simulink model "solar_wind_system_with_statcom"  (R2024a)
settings: Solver=VariableStepAuto  StartTime=0.0  StopTime=1  RelTol=1e-3
undefined symbols (not defined in the file): DiscIntNeverNeededParam, R
libraries: neural x24, spsSeriesRLCBranchLib x24, spsVoltageMeasurementLib x12, spsDiodeLib x10, powerlib_extras x9, simulink x7, spsIGBTDiodeLib x6, spsCurrentMeasurementLib x5, spsThreePhaseVIMeasurementLib x4, spsBreakerLib x3, spsPower3phInstantaneousLib x3, spsControlledCurrentSourceLib x3
(part 1 of 3)
settings Model: Creator=prabh  LastModifiedBy=HP

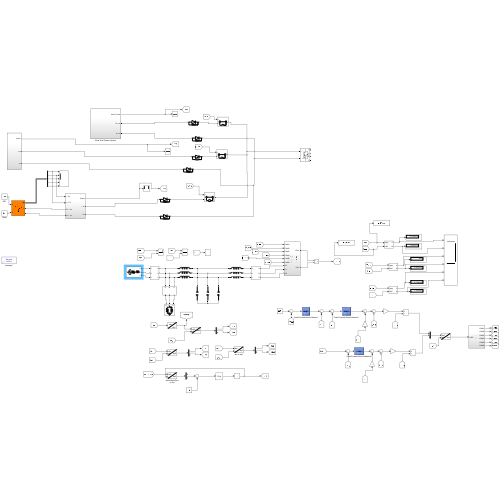
[thumbnail: Simulink's stored preview of the top-level diagram]
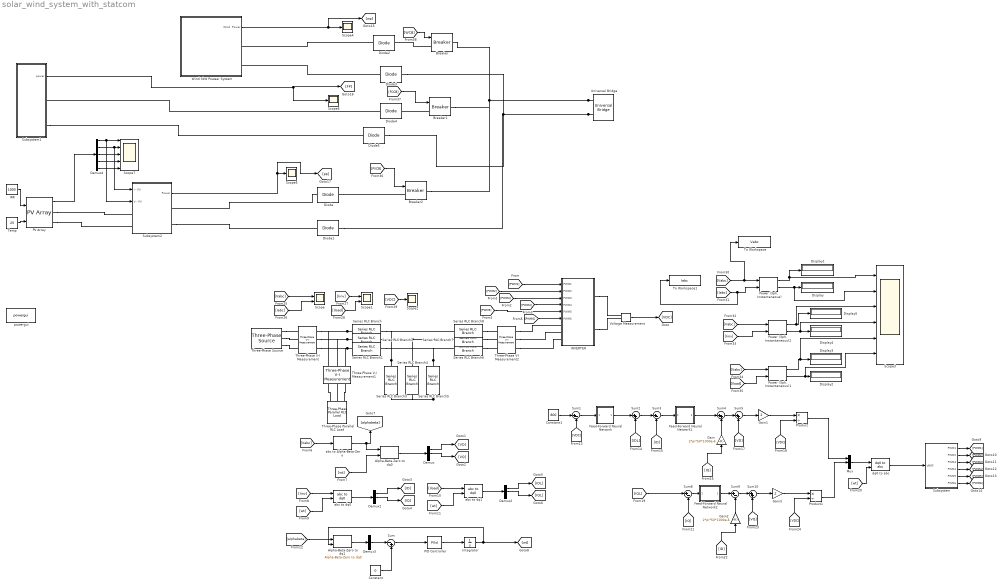
== system solar_wind_system_with_statcom ==
  Alpha-Beta-Zero to dq0 : spsAlphaBetaZerotodq0Lib/Alpha-Beta-Zero to dq0  Alignment=90 degrees behind phase A axis
  Alpha-Beta-Zero to dq1 : spsAlphaBetaZerotodq0Lib/Alpha-Beta-Zero to dq0  Alignment=90 degrees behind phase A axis
  Breaker : spsBreakerLib/Breaker  InitialState=1  SwitchingTimes="[1/60  5/60]"  External=on  BreakerResistance=0.01  SnubberResistance=1e6  SnubberCapacitance=inf  Measurements=None  MoreParameters=on  NoBreakLoop=off
  Breaker1 : spsBreakerLib/Breaker  InitialState=1  SwitchingTimes="[1/60  5/60]"  External=on  BreakerResistance=0.01  SnubberResistance=1e6  SnubberCapacitance=inf  Measurements=None  MoreParameters=on  NoBreakLoop=off
  Breaker2 : spsBreakerLib/Breaker  InitialState=1  SwitchingTimes="[1/60  5/60]"  External=on  BreakerResistance=0.01  SnubberResistance=1e6  SnubberCapacitance=inf  Measurements=None  MoreParameters=on  NoBreakLoop=off
  Constant : Constant  Value=0
  Constant1 : Constant  Value=800
  Demux{,1..3} (4 alike) : Demux  Outputs=3
  Demux4 : Demux  Outputs=5
  Diode{,1..5} (6 alike) : spsDiodeLib/Diode  Ron=0.001  Lon=0  Vf=0.8  IC=0  UseSnubber=off  Rs=500  Cs=250e-9  Measurements=off
  Display{,1..5} (6 alike) : Display
  Feed-Forward Neural Network : Subsystem
      mask help: Feed-Forward Neural Network
      mask Display: e = 0.06;c1 = [120 150 230]/255;c2 = ([120 150 230]+0)/383;c3 = ([120 150 230]+128)/383;patch([0 1 1 0],[0 0 1 1],c1);patch([0 1 1 1-e 1-e 0+e],[0 0 1 1-e 0+e 0+e],c2);patch([0 0 1 1-e 0+e 0+e],[0 1 1 1-e 1-e 0+e],c3);plot([0 1 1 0 0],[0 0 1 1 0]);fprintf('NNET');port_label('input',1,' Input');port_label('output',1,'Output ');
  Feed-Forward Neural Network1 : Subsystem
      mask help: Feed-Forward Neural Network
      mask Display: e = 0.06;c1 = [120 150 230]/255;c2 = ([120 150 230]+0)/383;c3 = ([120 150 230]+128)/383;patch([0 1 1 0],[0 0 1 1],c1);patch([0 1 1 1-e 1-e 0+e],[0 0 1 1-e 0+e 0+e],c2);patch([0 0 1 1-e 0+e 0+e],[0 1 1 1-e 1-e 0+e],c3);plot([0 1 1 0 0],[0 0 1 1 0]);fprintf('NNET');port_label('input',1,' Input');port_label('output',1,'Output ');
  Feed-Forward Neural Network2 : Subsystem
      mask help: Feed-Forward Neural Network
      mask Display: e = 0.06;c1 = [120 150 230]/255;c2 = ([120 150 230]+0)/383;c3 = ([120 150 230]+128)/383;patch([0 1 1 0],[0 0 1 1],c1);patch([0 1 1 1-e 1-e 0+e],[0 0 1 1-e 0+e 0+e],c2);patch([0 0 1 1-e 0+e 0+e],[0 1 1 1-e 1-e 0+e],c3);plot([0 1 1 0 0],[0 0 1 1 0]);fprintf('NNET');port_label('input',1,' Input');port_label('output',1,'Output ');
  Gain : Gain  Gain=2*pi*50*1000e-6
  Gain1 : Gain  Gain=2
  Gain2 : Gain  Gain=2*pi*50*1000e-6
  Gain3 : Gain  Gain=2
  INVERTER : Subsystem
  IRR : Constant  Value=1000
  Integrator : Integrator
  Mux : Mux  Inputs=3
  PID Controller : slpidlib/PID Controller  Controller=PI  Form=Parallel  TimeDomain=Continuous-time  UseExternalTs=off  SampleTime=-1  IntegratorMethod=Forward Euler  FilterMethod=Forward Euler  ControllerParametersSource=internal  P=10  I=50000  UseKiTs=off  D=0  UseExternalDerivativeSource=off  N=100  UseFilter=on  TunerSelectOption=Transfer Function Based (PID Tuner App)  InitialConditionSource=internal  InitialConditionForIntegrator=0  InitialConditionForFilter=0  DifferentiatorICPrevScaledInput=0  ExternalReset=none  TrackingMode=off  Kt=1  LimitOutput=off  SatLimitsSource=internal  UpperSaturationLimit=inf  LowerSaturationLimit=-inf  LinearizeAsGain=on  AntiWindupMode=none  Kb=1  LimitIntegrator=off  UpperIntegratorSaturationLimit=inf  LowerIntegratorSaturationLimit=-inf  POutMin=[]  POutMax=[]  IOutMin=[]  IOutMax=[]  DOutMin=[]  DOutMax=[]  NOutMin=[]  NOutMax=[]  SumOutMin=[]  SumOutMax=[]  SaturationOutMin=[]  SaturationOutMax=[]  PParamMin=[]  PParamMax=[]  IParamMin=[]  IParamMax=[]  DParamMin=[]  DParamMax=[]  NParamMin=[]  NParamMax=[]  KbParamMin=[]  KbParamMax=[]  KtParamMin=[]  KtParamMax=[]  KbOutMin=[]  KbOutMax=[]  KtOutMin=[]  KtOutMax=[]  IntegratorOutMin=[]  IntegratorOutMax=[]  FilterOutMin=[]  FilterOutMax=[]  SumI1OutMin=[]  SumI1OutMax=[]  SumI2OutMin=[]  SumI2OutMax=[]  SumI3OutMin=[]  SumI3OutMax=[]  SumI4OutMin=[]  SumI4OutMax=[]  SumDOutMin=[]  SumDOutMax=[]  DifferentiatorOutMin=[]  DifferentiatorOutMax=[]  FilterDiffOutCoefMin=[]  FilterDiffOutCoefMax=[]  ReciprocalOutMin=[]  ReciprocalOutMax=[]  SumDenOutMin=[]  SumDenOutMax=[]  SumNumOutMin=[]  SumNumOutMax=[]  DivideOutMin=[]  DivideOutMax=[]  UdiffTsProdOutMin=[]  UdiffTsProdOutMax=[]  NTsProdOutMin=[]  NTsProdOutMax=[]  UintegralTsProdOutMin=[]  UintegralTsProdOutMax=[]  UngainTsProdOutMin=[]  UngainTsProdOutMax=[]  ClampingZeroOutDataTypeStr=Inherit: Inherit via back propagation  ClampingZeroOutMin=[]  ClampingZeroOutMax=[]  FilterDenConstantOutDataTypeStr=Inherit: Inherit via back propagation  FilterDenConstantOutMin=[]  FilterDenConstantOutMax=[]  PCopyOutDataTypeStr=Inherit: Inherit via back propagation  PCopyOutMin=[]  PCopyOutMax=[]  NCopyOutDataTypeStr=Inherit: Inherit via back propagation  NCopyOutMin=[]  NCopyOutMax=[]  IntegratorContinuousStateAttributes=''  IntegratorStateMustResolveToSignalObject=off  IntegratorRTWStateStorageClass=Auto  FilterContinuousStateAttributes=''  FilterStateMustResolveToSignalObject=off  FilterRTWStateStorageClass=Auto  ParallelPVariant=InternalParameters  IdealPVariant=Disabled  IVariant=InternalParameters  DVariant=Disabled  IntegratorVariant=Continuous  SatVariant=Disabled  AWVariant=Passthrough  PCopyVariant=Disabled  TRVariant=Disabled  FdbkBlocksVariant=Forward  IdealPFdbkVariant=Disabled  SatFdbkVariant=Disabled  DerivativeFilterVariant=Disabled  NVariant=Disabled  NCopyVariant=Disabled_SignalSpec  FilterICVariant=Disabled  IntegratorICVariant=InternalICs  ExternalResetVariant=Disabled  TRSumVariant=Passthrough  SumFdbkVariant=Disabled  SumVariant=Sum_PI  TsampFilterVariant=InternalTs  TsampNgainVariant=Passthrough  TsampIntegralVariant=Disabled_SignalSpec  ExternalSaturationOutDataTypeStr=Inherit: Same as second input  DerivativeSourceVariant=Disabled
  PV Array : spsPVArrayLib/PV Array  Npar=10  Nser=5  PlotType=array @ 25 deg.C & specified irradiances  S_vec="[ 1000  500  100 ]"  Temp_C_vec="[ 45 25  ]"  ModuleName=User-defined  PlotWhenSelected=off  Pm=334.905  Ncell=80  Voc=49.9  Isc=9  Vm=41.5  Im=8.07  beta_Voc_pc=-0.36  alpha_Isc_pc=0.09  beta_Voc=-0.17964  alpha_Isc=0.0081  IL=9.0297  I0=3.1312e-10  nI=1.0111  Rsh=77.6407  Rs=0.25633  RobustModel=off  RobustCellTemperature=313.3991  BAL=off  Tc=1e-6  Tfilter=5e-5
  "Power (3ph, Instantaneous)" : spsPower3phInstantaneousLib/Power (3ph, Instantaneous)
  "Power (3ph, Instantaneous)1" : spsPower3phInstantaneousLib/Power (3ph, Instantaneous)
  "Power (3ph, Instantaneous)2" : spsPower3phInstantaneousLib/Power (3ph, Instantaneous)
  Product : Product  Inputs=*/
  Product1 : Product  Inputs=*/
  Scope : Scope  NumInputPorts=2
  Scope1 : Scope  NumInputPorts=2
  Scope{2,4..6} (4 alike) : Scope
  Scope3 : Scope  NumInputPorts=6
  Scope7 : Scope  NumInputPorts=5
  Series RLC Branch{,1..2,6..8} (6 alike) : spsSeriesRLCBranchLib/Series RLC Branch  LConnTagsString=__new0  RConnTagsString=__new0  BranchType=L  Resistance=1  Inductance=500e-6  SetiL0=off  InitialCurrent=0  Capacitance=1e-6  Setx0=off  InitialVoltage=0  Measurements=None
  Series RLC Branch3 : spsSeriesRLCBranchLib/Series RLC Branch  LConnTagsString=__new0  RConnTagsString=__new0  BranchType=C  Resistance=1  Inductance=500e-6  SetiL0=off  InitialCurrent=0  Capacitance=100e-6  Setx0=off  InitialVoltage=0  Measurements=None
  Series RLC Branch4 : spsSeriesRLCBranchLib/Series RLC Branch  LConnTagsString=__new0  RConnTagsString=__new0  BranchType=C  Resistance=1  Inductance=500e-6  SetiL0=off  InitialCurrent=0  Capacitance=100e-6  Setx0=off  InitialVoltage=0  Measurements=None
  Series RLC Branch5 : spsSeriesRLCBranchLib/Series RLC Branch  LConnTagsString=__new0  RConnTagsString=__new0  BranchType=C  Resistance=1  Inductance=500e-6  SetiL0=off  InitialCurrent=0  Capacitance=100e-6  Setx0=off  InitialVoltage=0  Measurements=None
  Subsystem : Subsystem
  Subsystem1 : Subsystem
  Subsystem2 : Subsystem
  Sum : Sum  Inputs=|-+
  Sum{1,3,8..9} (4 alike) : Sum  Inputs=|+-
  Sum{2,4..5,10} (4 alike) : Sum  Inputs=|++
  "Temp " : Constant  Value=25
  Three-Phase Parallel RLC Load : spsThreePhaseParallelRLCLoadLib/Three-Phase Parallel RLC Load  LConnTagsString=A|B|C  Configuration=Y (grounded)  NominalVoltage=415  Vabc=[1e3 1e3 1e3]  Vabcp=[1e3 1e3 1e3]  NominalFrequency=50  UnbalancedPower=off  ActivePower=150000  InductivePower=75000  CapacitivePower=0  Pabc=[10e3 9e3 11e3]  QLabc=[100 90 110]  QCabc=[100 90 110]  Pabcp=[10e3 9e3 11e3]  QLabcp=[100 90 110]  QCabcp=[100 90 110]  Measurements=None  LoadType=constant Z
  Three-Phase V-I Measurement : spsThreePhaseVIMeasurementLib/Three-Phase V-I Measurement  VoltageMeasurement=phase-to-ground  SetLabelV=on  LabelV=Vabc  Vpu=off  VpuLL=off  CurrentMeasurement=yes  SetLabelI=on  LabelI=Iabc  Ipu=off  Pbase=100e6  Vbase=500e3  OutputType=Complex  PhasorSimulation=off  PSBequivalent=0
  Three-Phase V-I Measurement1 : spsThreePhaseVIMeasurementLib/Three-Phase V-I Measurement  VoltageMeasurement=phase-to-ground  SetLabelV=on  LabelV=Vload  Vpu=off  VpuLL=off  CurrentMeasurement=yes  SetLabelI=on  LabelI=Iload  Ipu=off  Pbase=100e6  Vbase=500e3  OutputType=Complex  PhasorSimulation=off  PSBequivalent=0
  Three-Phase V-I Measurement2 : spsThreePhaseVIMeasurementLib/Three-Phase V-I Measurement  VoltageMeasurement=phase-to-ground  SetLabelV=on  LabelV=Vinv  Vpu=off  VpuLL=off  CurrentMeasurement=yes  SetLabelI=on  LabelI=Iinv  Ipu=off  Pbase=100e6  Vbase=500e3  OutputType=Complex  PhasorSimulation=off  PSBequivalent=0
  Three-Phase Source : spsThreePhaseSourceLib/Three-Phase Source  InternalConnection=Y  VoltagePhases=off  Voltage=500  PhaseAngle=0  Voltage_phases=[25e3 25e3 25e3]/sqrt(3)  PhaseAngles_phases=[0 -120 +120]  Frequency=50  NonIdealSource=on  SpecifyImpedance=off  Resistance=1e-6  Inductance=1e-6  ShortCircuitLevel=100e6  BaseVoltage=415  XRratio=7  BusType=swing  Pref=10e3  Qref=0  Prefabc=[10e3, 10e3, 10e3]  Qrefabc=[0, 0, 0]  Qmin=-inf  Qmax=inf
  To Workspace : ToWorkspace  VariableName=Vabc  SampleTime=-1
  To Workspace1 : ToWorkspace  VariableName=Iabc  SampleTime=-1
  Universal Bridge : spsUniversalBridgeLib/Universal Bridge  Arms=3  SnubberResistance=1e5  SnubberCapacitance=inf  Device=MOSFET / Diodes  Ron=1e-3  Lon=0  ForwardVoltages="[  0  0  ]"  ForwardVoltage=0  GTOparameters=[ 10e-6 , 20e-6 ]  IGBTparameters=[ 1e-6 , 2e-6 ]  Measurements=None  Measurements_2=None  converterType=Rectifier
  Voltage Measurement : spsVoltageMeasurementLib/Voltage Measurement  PhasorSimulation=off  OutputType=Complex  PSBequivalent=0
  Wind 3kW Poweer System : Subsystem
  abc to Alpha-Beta-Zero : spsabctoAlphaBetaZeroLib/abc to Alpha-Beta-Zero
  abc to dq0 : spsabctodq0Lib/abc to dq0  Alignment=90 degrees behind phase A axis
  abc to dq1 : spsabctodq0Lib/abc to dq0  Alignment=90 degrees behind phase A axis
  dq0 to abc : spsdq0toabcLib/dq0 to abc  Alignment=90 degrees behind phase A axis
  powergui : sps_lib/powergui  Priority=1  SimulationMode=Discrete  SampleTime=1e-6  frequency=60  Iterations=50  frequencyindice=0  Pbase=100e6  ErrMax=1e-4  UnitsV=kV  UnitsW=MW  buscounter=0  FunctionMessages=off  echomessages=off  EnableUseOfTLC=off  CurrentSourceSwitches=off  DisableSnubberDevices=off  DisableRonSwitches=off  DisableVfSwitches=off  DisplayEquations=off  AutomaticDiscreteSolvers=off  SolverType=Tustin/Backward Euler (TBE)  Interpol=off  ExternalGateDelay=off  methode=off  Ts=100  x0status=blocks  SPID=on  SwTol=0  HookPort=off  NonlinearTolerance=1e-4  nMaxIteration=100  ContinueOnMaxIteration=off  RestoreLinks=warning  ResistiveCurrentMeasurement=off  Frange=[0:2:500]  Ylog=off  Xlog=on  ShowGrid=off  save=off  variable=ZData  structure=0  ZoomFFT=off  StartTime=0.0  cycles=1  DisplayStyle=1  fundamental=60  FreqAxis=off  MaxFrequency=1000  frequencyindicesteady=1  RmsSteady=1  display=off
  wires:
  [Iload] -> "Power (3ph, Instantaneous)1"/2
  [PWM3] -> INVERTER/3(PWM3)
  [Vabc] -> "Power (3ph, Instantaneous)1"/1
  [Iload] -> Scope1/2
  Sum1/1 -> Feed-Forward Neural Network/1(Input)
  [IQL] -> Sum8/1
  [Iabc] -> To Workspace1/1, "Power (3ph, Instantaneous)"/2
  Demux2/2 -> [IQL]
  "Power (3ph, Instantaneous)2"/1 -> Scope3/3, Display5/1
  "Power (3ph, Instantaneous)1"/2 -> Scope3/6, Display2/1
  Integrator/1 -> Alpha-Beta-Zero to dq1/2, [wt]
  Sum3/1 -> Feed-Forward Neural Network1/1(Input)
  [Iinv] -> "Power (3ph, Instantaneous)2"/2
  Demux3/2 -> Sum/1
  "Power (3ph, Instantaneous)2"/2 -> Scope3/4, Display4/1
  [Iinv] -> Scope1/1
  Demux/2 -> [VQ]
  abc to Alpha-Beta-Zero/1 -> [alphabeta], Alpha-Beta-Zero to dq0/1
  [Vabc] -> To Workspace/1, "Power (3ph, Instantaneous)"/1
  "Power (3ph, Instantaneous)"/1 -> Scope3/1, Display1/1
  Alpha-Beta-Zero to dq1/1 -> Demux3/1
  Subsystem/6(PWM6) -> [PWM6]
  Demux1/2 -> [IQ]
  Subsystem/3(PWM3) -> [PWM3]
  Feed-Forward Neural Network2/1(Output) -> Sum9/1
  [Iinv] -> abc to dq0/1
  Subsystem/1(PWM1) -> [PWM1]
  [IQ] -> Sum8/2
  [Iabc] -> Scope/2
  Gain/1 -> Sum4/2
  Sum/1 -> PID Controller/1
  Subsystem/4(PWM4) -> [PWM4]
  [wt] -> dq0 to abc/2
  Voltage Measurement/1 -> [VDC]
  [VDC] -> Scope2/1
  Sum8/1 -> Feed-Forward Neural Network2/1(Input)
  [Vabc] -> Scope/1
  Mux/1 -> dq0 to abc/1
  Sum4/1 -> Sum5/1
  Product1/1 -> Mux/2
  Gain2/1 -> Sum9/2
  Sum9/1 -> Sum10/1
  Product/1 -> Mux/1
  [VQ] -> Sum10/2
  [ID] -> Sum3/2
  Gain1/1 -> Product/1
  [VD] -> Sum5/2
  Sum5/1 -> Gain1/1
  [alphabeta] -> Alpha-Beta-Zero to dq1/1
  Subsystem/2(PWM2) -> [PWM2]
  Sum2/1 -> Sum3/1
  [IQ] -> Gain/1
  [IDL] -> Sum2/2
  Gain3/1 -> Product1/1
  [Iload] -> abc to dq1/1
  [VDC] -> Sum1/2
  [Vabc] -> abc to Alpha-Beta-Zero/1
  PID Controller/1 -> Integrator/1
  [PWM5] -> INVERTER/5(PWM5)
  Subsystem/5(PWM5) -> [PWM5]
  [wt] -> abc to dq1/2
  [PWM2] -> INVERTER/2(PWM2)
  Demux1/1 -> [ID]
  [wt] -> abc to dq0/2
  [ID] -> Gain2/1
  [PWM1] -> INVERTER/1(PWM1)
  [wt] -> Alpha-Beta-Zero to dq0/2
  [VDC] -> Product1/2
  Demux2/1 -> [IDL]
  abc to dq0/1 -> Demux1/1
  dq0 to abc/1 -> Subsystem/1(VREF)
  Constant1/1 -> Sum1/1
  Alpha-Beta-Zero to dq0/1 -> Demux/1
  [PWM6] -> INVERTER/6(PWM6)
  Sum10/1 -> Gain3/1
  [Vabc] -> "Power (3ph, Instantaneous)2"/1
  "Power (3ph, Instantaneous)1"/1 -> Scope3/5, Display3/1
  [VDC] -> Product/2
  Feed-Forward Neural Network/1(Output) -> Sum2/1
  abc to dq1/1 -> Demux2/1
  Feed-Forward Neural Network1/1(Output) -> Sum4/1
  "Power (3ph, Instantaneous)"/2 -> Scope3/2, Display/1
  [PWM4] -> INVERTER/4(PWM4)
  Constant/1 -> Sum/2
  Demux/1 -> [VD]
  "Temp "/1 -> PV Array/2
  [PVCB] -> Breaker2/1
  Demux4/4 -> Scope7/4
  Subsystem1/1(power) -> [FP], Scope6/1
  Wind 3kW Poweer System/1(Wind  Power) -> [wp], Scope4/1
  Demux4/2 -> Scope7/2, Subsystem2/1(I - PV)
  IRR/1 -> PV Array/1
  [WCB] -> Breaker/1
  Subsystem2/1(Power) -> [pp], Scope5/1
  Demux4/1 -> Scope7/1, Subsystem2/2(V - PV)
  Demux4/5 -> Scope7/5
  Demux4/3 -> Scope7/3
  PV Array/1 -> Demux4/1
  [FCCB] -> Breaker1/1
  connections:
  Series RLC Branch2/LConn1 -- Three-Phase V-I Measurement/RConn3 -- Three-Phase V-I Measurement1/LConn3
  Series RLC Branch5/RConn1 -- Series RLC Branch3/RConn1 -- Series RLC Branch4/RConn1
  Series RLC Branch3/LConn1 -- Series RLC Branch8/LConn1 -- Series RLC Branch/RConn1
  Series RLC Branch7/LConn1 -- Series RLC Branch1/RConn1 -- Series RLC Branch4/LConn1
  Series RLC Branch1/LConn1 -- Three-Phase V-I Measurement/RConn2 -- Three-Phase V-I Measurement1/LConn2
  Series RLC Branch/LConn1 -- Three-Phase V-I Measurement/RConn1 -- Three-Phase V-I Measurement1/LConn1
  Series RLC Branch5/LConn1 -- Series RLC Branch6/LConn1 -- Series RLC Branch2/RConn1
  Three-Phase V-I Measurement2/LConn2 -- INVERTER/LConn2
  Series RLC Branch6/RConn1 -- Three-Phase V-I Measurement2/RConn3
  Three-Phase V-I Measurement2/LConn3 -- INVERTER/LConn3
  Three-Phase Source/RConn1 -- Three-Phase V-I Measurement/LConn1
  INVERTER/RConn2 -- Voltage Measurement/LConn2
  Three-Phase Parallel RLC Load/LConn2 -- Three-Phase V-I Measurement1/RConn2
  Series RLC Branch8/RConn1 -- Three-Phase V-I Measurement2/RConn1
  Three-Phase Parallel RLC Load/LConn3 -- Three-Phase V-I Measurement1/RConn3
  Series RLC Branch7/RConn1 -- Three-Phase V-I Measurement2/RConn2
  INVERTER/RConn1 -- Voltage Measurement/LConn1
  Three-Phase Parallel RLC Load/LConn1 -- Three-Phase V-I Measurement1/RConn1
  Three-Phase Source/RConn2 -- Three-Phase V-I Measurement/LConn2
  Three-Phase Source/RConn3 -- Three-Phase V-I Measurement/LConn3
  Three-Phase V-I Measurement2/LConn1 -- INVERTER/LConn1
  Universal Bridge/RConn2 -- Diode3/RConn1 -- Diode5/RConn1 -- Diode1/RConn1
  Universal Bridge/RConn1 -- Breaker/RConn1 -- Breaker2/RConn1 -- Breaker1/RConn1
  Diode2/LConn1 -- Wind 3kW Poweer System/RConn1
  Subsystem2/RConn2 -- Diode1/LConn1
  Subsystem1/RConn2 -- Diode5/LConn1
  PV Array/RConn1 -- Subsystem2/LConn1
  Breaker2/LConn1 -- Diode/RConn1
  Diode4/LConn1 -- Subsystem1/RConn1
  Breaker/LConn1 -- Diode2/RConn1
  Breaker1/LConn1 -- Diode4/RConn1
  PV Array/RConn2 -- Subsystem2/LConn2
  Diode3/LConn1 -- Wind 3kW Poweer System/RConn2
  Diode/LConn1 -- Subsystem2/RConn1

== system solar_wind_system_with_statcom/Feed-Forward Neural Network ==
  Input : Inport  PortDimensions=1
      mask Display: e = 0.06;c1 = [120 230 180]/255;c2 = ([120 230 180]+0)/(256+128);c3 = ([120 230 180]+128)/(256+128);patch([0 1 1 0],[0 0 1 1],c1);patch([0 1 1 1-e 1-e 0+e],[0 0 1 1-e 0+e 0+e],c2);patch([0 0 1 1-e 0+e 0+e],[0 1 1 1-e 1-e 0+e],c3);plot([0 1 1 0 0],[0 0 1 1 0]);
  Layer 1 : Subsystem
      mask Display: e = 0.06;c1 = [120 150 230]/255;c2 = ([120 150 230]+0)/383;c3 = ([120 150 230]+128)/383;patch([0 1 1 0],[0 0 1 1],c1);patch([0 1 1 1-e 1-e 0+e],[0 0 1 1-e 0+e 0+e],c2);patch([0 0 1 1-e 0+e 0+e],[0 1 1 1-e 1-e 0+e],c3);plot([0 1 1 0 0],[0 0 1 1 0]);
  Layer 2 : Subsystem
      mask Display: e = 0.06;c1 = [120 150 230]/255;c2 = ([120 150 230]+0)/383;c3 = ([120 150 230]+128)/383;patch([0 1 1 0],[0 0 1 1],c1);patch([0 1 1 1-e 1-e 0+e],[0 0 1 1-e 0+e 0+e],c2);patch([0 0 1 1-e 0+e 0+e],[0 1 1 1-e 1-e 0+e],c3);plot([0 1 1 0 0],[0 0 1 1 0]);
  Process Input 1 : Subsystem
      mask Display: e = 0.06;c1 = [120 150 230]/255;c2 = ([120 150 230]+0)/383;c3 = ([120 150 230]+128)/383;patch([0 1 1 0],[0 0 1 1],c1);patch([0 1 1 1-e 1-e 0+e],[0 0 1 1-e 0+e 0+e],c2);patch([0 0 1 1-e 0+e 0+e],[0 1 1 1-e 1-e 0+e],c3);plot([0 1 1 0 0],[0 0 1 1 0]);
  Process Output 1 : Subsystem
      mask Display: e = 0.06;c1 = [120 150 230]/255;c2 = ([120 150 230]+0)/383;c3 = ([120 150 230]+128)/383;patch([0 1 1 0],[0 0 1 1],c1);patch([0 1 1 1-e 1-e 0+e],[0 0 1 1-e 0+e 0+e],c2);patch([0 0 1 1-e 0+e 0+e],[0 1 1 1-e 1-e 0+e],c3);plot([0 1 1 0 0],[0 0 1 1 0]);
  Output : Outport  InitialOutput=0
      mask Display: e = 0.06;c1 = [120 230 180]/255;c2 = ([120 230 180]+0)/(256+128);c3 = ([120 230 180]+128)/(256+128);patch([0 1 1 0],[0 0 1 1],c1);patch([0 1 1 1-e 1-e 0+e],[0 0 1 1-e 0+e 0+e],c2);patch([0 0 1 1-e 0+e 0+e],[0 1 1 1-e 1-e 0+e],c3);plot([0 1 1 0 0],[0 0 1 1 0]);
  wires:
  Input/1 -> Process Input 1/1(x)
  Process Output 1/1(y) -> Output/1
  Process Input 1/1(p) -> Layer 1/1("p{1}")
  Layer 1/1("a{1}") -> [feedback1]
  [feedback1] -> Layer 2/1("a{1} ")
  Layer 2/1("a{2}") -> Process Output 1/1(a)

== system solar_wind_system_with_statcom/Feed-Forward Neural Network1 ==
  Input : Inport  PortDimensions=1
      mask Display: e = 0.06;c1 = [120 230 180]/255;c2 = ([120 230 180]+0)/(256+128);c3 = ([120 230 180]+128)/(256+128);patch([0 1 1 0],[0 0 1 1],c1);patch([0 1 1 1-e 1-e 0+e],[0 0 1 1-e 0+e 0+e],c2);patch([0 0 1 1-e 0+e 0+e],[0 1 1 1-e 1-e 0+e],c3);plot([0 1 1 0 0],[0 0 1 1 0]);
  Layer 1 : Subsystem
      mask Display: e = 0.06;c1 = [120 150 230]/255;c2 = ([120 150 230]+0)/383;c3 = ([120 150 230]+128)/383;patch([0 1 1 0],[0 0 1 1],c1);patch([0 1 1 1-e 1-e 0+e],[0 0 1 1-e 0+e 0+e],c2);patch([0 0 1 1-e 0+e 0+e],[0 1 1 1-e 1-e 0+e],c3);plot([0 1 1 0 0],[0 0 1 1 0]);
  Layer 2 : Subsystem
      mask Display: e = 0.06;c1 = [120 150 230]/255;c2 = ([120 150 230]+0)/383;c3 = ([120 150 230]+128)/383;patch([0 1 1 0],[0 0 1 1],c1);patch([0 1 1 1-e 1-e 0+e],[0 0 1 1-e 0+e 0+e],c2);patch([0 0 1 1-e 0+e 0+e],[0 1 1 1-e 1-e 0+e],c3);plot([0 1 1 0 0],[0 0 1 1 0]);
  Process Input 1 : Subsystem
      mask Display: e = 0.06;c1 = [120 150 230]/255;c2 = ([120 150 230]+0)/383;c3 = ([120 150 230]+128)/383;patch([0 1 1 0],[0 0 1 1],c1);patch([0 1 1 1-e 1-e 0+e],[0 0 1 1-e 0+e 0+e],c2);patch([0 0 1 1-e 0+e 0+e],[0 1 1 1-e 1-e 0+e],c3);plot([0 1 1 0 0],[0 0 1 1 0]);
  Process Output 1 : Subsystem
      mask Display: e = 0.06;c1 = [120 150 230]/255;c2 = ([120 150 230]+0)/383;c3 = ([120 150 230]+128)/383;patch([0 1 1 0],[0 0 1 1],c1);patch([0 1 1 1-e 1-e 0+e],[0 0 1 1-e 0+e 0+e],c2);patch([0 0 1 1-e 0+e 0+e],[0 1 1 1-e 1-e 0+e],c3);plot([0 1 1 0 0],[0 0 1 1 0]);
  Output : Outport  InitialOutput=0
      mask Display: e = 0.06;c1 = [120 230 180]/255;c2 = ([120 230 180]+0)/(256+128);c3 = ([120 230 180]+128)/(256+128);patch([0 1 1 0],[0 0 1 1],c1);patch([0 1 1 1-e 1-e 0+e],[0 0 1 1-e 0+e 0+e],c2);patch([0 0 1 1-e 0+e 0+e],[0 1 1 1-e 1-e 0+e],c3);plot([0 1 1 0 0],[0 0 1 1 0]);
  wires:
  Input/1 -> Process Input 1/1(x)
  Process Output 1/1(y) -> Output/1
  Process Input 1/1(p) -> Layer 1/1("p{1}")
  Layer 1/1("a{1}") -> [feedback1]
  [feedback1] -> Layer 2/1("a{1} ")
  Layer 2/1("a{2}") -> Process Output 1/1(a)

== system solar_wind_system_with_statcom/Feed-Forward Neural Network2 ==
  Input : Inport  PortDimensions=1
      mask Display: e = 0.06;c1 = [120 230 180]/255;c2 = ([120 230 180]+0)/(256+128);c3 = ([120 230 180]+128)/(256+128);patch([0 1 1 0],[0 0 1 1],c1);patch([0 1 1 1-e 1-e 0+e],[0 0 1 1-e 0+e 0+e],c2);patch([0 0 1 1-e 0+e 0+e],[0 1 1 1-e 1-e 0+e],c3);plot([0 1 1 0 0],[0 0 1 1 0]);
  Layer 1 : Subsystem
      mask Display: e = 0.06;c1 = [120 150 230]/255;c2 = ([120 150 230]+0)/383;c3 = ([120 150 230]+128)/383;patch([0 1 1 0],[0 0 1 1],c1);patch([0 1 1 1-e 1-e 0+e],[0 0 1 1-e 0+e 0+e],c2);patch([0 0 1 1-e 0+e 0+e],[0 1 1 1-e 1-e 0+e],c3);plot([0 1 1 0 0],[0 0 1 1 0]);
  Layer 2 : Subsystem
      mask Display: e = 0.06;c1 = [120 150 230]/255;c2 = ([120 150 230]+0)/383;c3 = ([120 150 230]+128)/383;patch([0 1 1 0],[0 0 1 1],c1);patch([0 1 1 1-e 1-e 0+e],[0 0 1 1-e 0+e 0+e],c2);patch([0 0 1 1-e 0+e 0+e],[0 1 1 1-e 1-e 0+e],c3);plot([0 1 1 0 0],[0 0 1 1 0]);
  Process Input 1 : Subsystem
      mask Display: e = 0.06;c1 = [120 150 230]/255;c2 = ([120 150 230]+0)/383;c3 = ([120 150 230]+128)/383;patch([0 1 1 0],[0 0 1 1],c1);patch([0 1 1 1-e 1-e 0+e],[0 0 1 1-e 0+e 0+e],c2);patch([0 0 1 1-e 0+e 0+e],[0 1 1 1-e 1-e 0+e],c3);plot([0 1 1 0 0],[0 0 1 1 0]);
  Process Output 1 : Subsystem
      mask Display: e = 0.06;c1 = [120 150 230]/255;c2 = ([120 150 230]+0)/383;c3 = ([120 150 230]+128)/383;patch([0 1 1 0],[0 0 1 1],c1);patch([0 1 1 1-e 1-e 0+e],[0 0 1 1-e 0+e 0+e],c2);patch([0 0 1 1-e 0+e 0+e],[0 1 1 1-e 1-e 0+e],c3);plot([0 1 1 0 0],[0 0 1 1 0]);
  Output : Outport  InitialOutput=0
      mask Display: e = 0.06;c1 = [120 230 180]/255;c2 = ([120 230 180]+0)/(256+128);c3 = ([120 230 180]+128)/(256+128);patch([0 1 1 0],[0 0 1 1],c1);patch([0 1 1 1-e 1-e 0+e],[0 0 1 1-e 0+e 0+e],c2);patch([0 0 1 1-e 0+e 0+e],[0 1 1 1-e 1-e 0+e],c3);plot([0 1 1 0 0],[0 0 1 1 0]);
  wires:
  Input/1 -> Process Input 1/1(x)
  Process Output 1/1(y) -> Output/1
  Process Input 1/1(p) -> Layer 1/1("p{1}")
  Layer 1/1("a{1}") -> [feedback1]
  [feedback1] -> Layer 2/1("a{1} ")
  Layer 2/1("a{2}") -> Process Output 1/1(a)

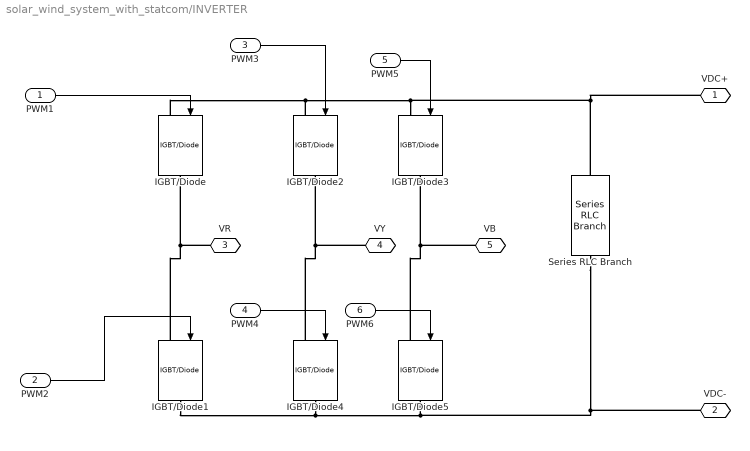
== system solar_wind_system_with_statcom/INVERTER ==
  PWM1 : Inport
  PWM2 : Inport  Port=2
  PWM3 : Inport  Port=3
  PWM4 : Inport  Port=4
  PWM5 : Inport  Port=5
  PWM6 : Inport  Port=6
  IGBT/Diode{,1..5} (6 alike) : spsIGBTDiodeLib/IGBT//Diode  Ron=1e-3  Rs=1e5  Cs=inf  Measurements=off
  Series RLC Branch : spsSeriesRLCBranchLib/Series RLC Branch  LConnTagsString=__new0  RConnTagsString=__new0  BranchType=RC  Resistance=1e-3  Inductance=1e-3  SetiL0=off  InitialCurrent=0  Capacitance=5600e-6  Setx0=off  InitialVoltage=0  Measurements=None
  VDC+ : PMIOPort  Side=Right
  VDC- : PMIOPort  Port=2  Side=Right
  VR : PMIOPort  Port=3  Side=Left
  VY : PMIOPort  Port=4  Side=Left
  VB : PMIOPort  Port=5  Side=Left
  wires:
  PWM6/1 -> IGBT/Diode5/1
  PWM5/1 -> IGBT/Diode3/1
  PWM1/1 -> IGBT/Diode/1
  PWM3/1 -> IGBT/Diode2/1
  PWM4/1 -> IGBT/Diode4/1
  PWM2/1 -> IGBT/Diode1/1
  connections:
  IGBT/Diode1/LConn1 -- VR/RConn1 -- IGBT/Diode/RConn1
  IGBT/Diode4/LConn1 -- VY/RConn1 -- IGBT/Diode2/RConn1
  IGBT/Diode1/RConn1 -- IGBT/Diode4/RConn1 -- VDC-/RConn1 -- Series RLC Branch/RConn1 -- IGBT/Diode5/RConn1
  IGBT/Diode/LConn1 -- IGBT/Diode2/LConn1 -- VDC+/RConn1 -- Series RLC Branch/LConn1 -- IGBT/Diode3/LConn1
  IGBT/Diode5/LConn1 -- VB/RConn1 -- IGBT/Diode3/RConn1

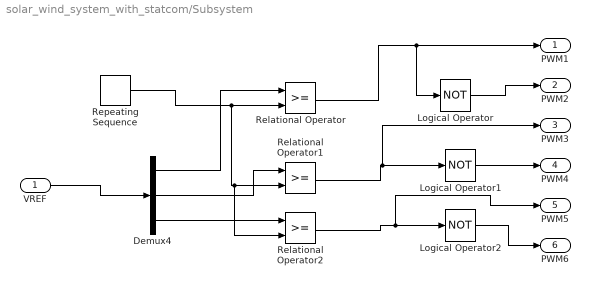
== system solar_wind_system_with_statcom/Subsystem ==
  VREF : Inport
  Demux4 : Demux  Outputs=3
  Logical Operator : Logic  Operator=NOT  AllPortsSameDT=off  OutDataTypeStr=boolean
  Logical Operator1 : Logic  Operator=NOT  AllPortsSameDT=off  OutDataTypeStr=boolean
  Logical Operator2 : Logic  Operator=NOT  AllPortsSameDT=off  OutDataTypeStr=boolean
  Relational Operator : RelationalOperator  OutDataTypeStr=boolean  RndMeth=Simplest  InputSameDT=off
  Relational Operator1 : RelationalOperator  OutDataTypeStr=boolean  RndMeth=Simplest  InputSameDT=off
  Relational Operator2 : RelationalOperator  OutDataTypeStr=boolean  RndMeth=Simplest  InputSameDT=off
  Repeating Sequence : simulink/Sources/Repeating Sequence  rep_seq_t=[0 0.00005 0.0001]  rep_seq_y=[-1 1 -1]
  PWM1 : Outport
  PWM2 : Outport  Port=2
  PWM3 : Outport  Port=3
  PWM4 : Outport  Port=4
  PWM5 : Outport  Port=5
  PWM6 : Outport  Port=6
  wires:
  Repeating Sequence/1 -> Relational Operator2/2, Relational Operator1/2, Relational Operator/2
  Demux4/3 -> Relational Operator2/1
  Logical Operator/1 -> PWM2/1
  VREF/1 -> Demux4/1
  Demux4/2 -> Relational Operator1/1
  Demux4/1 -> Relational Operator/1
  Relational Operator2/1 -> PWM5/1, Logical Operator2/1
  Logical Operator1/1 -> PWM4/1
  Relational Operator1/1 -> PWM3/1, Logical Operator1/1
  Relational Operator/1 -> PWM1/1, Logical Operator/1
  Logical Operator2/1 -> PWM6/1

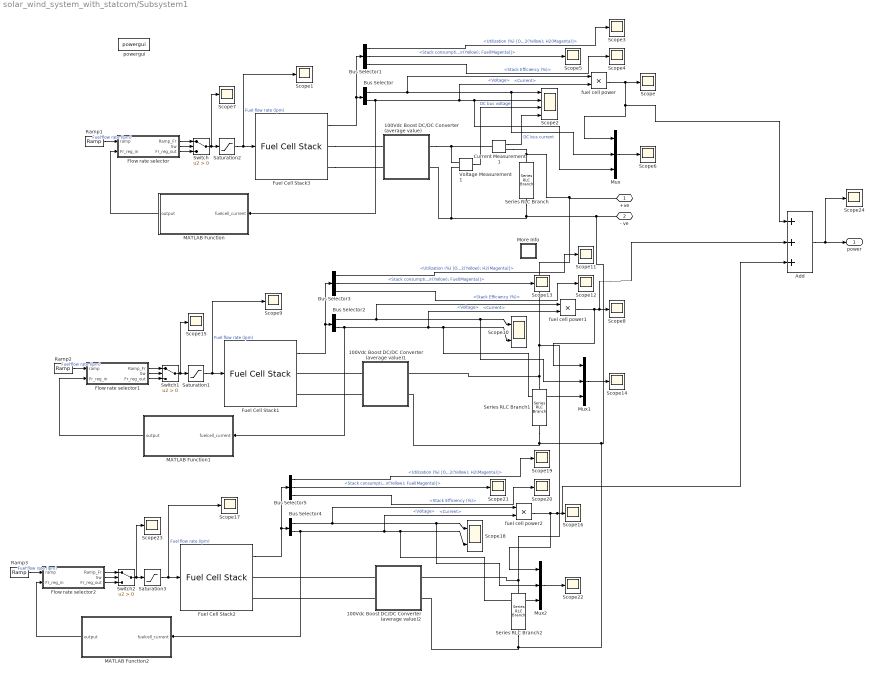
== system solar_wind_system_with_statcom/Subsystem1 ==
  100Vdc Boost DC/DC Converter (average value) : Subsystem
  100Vdc Boost DC/DC Converter (average value)1 : Subsystem
  100Vdc Boost DC/DC Converter (average value)2 : Subsystem
  Add : Sum  Inputs=+++
  Bus Selector : BusSelector  OutputSignals=Voltage,Current
  Bus Selector1 : BusSelector  OutputSignals=Utilization (%) [O2(Yellow); H2(Magenta)],Stack consumption (lpm) [Air(Yellow); Fuel(Magenta)],Stack Efficiency (%)
  Bus Selector2 : BusSelector  OutputSignals=Voltage,Current
  Bus Selector3 : BusSelector  OutputSignals=Utilization (%) [O2(Yellow); H2(Magenta)],Stack consumption (lpm) [Air(Yellow); Fuel(Magenta)],Stack Efficiency (%)
  Bus Selector4 : BusSelector  OutputSignals=Voltage,Current
  Bus Selector5 : BusSelector  OutputSignals=Utilization (%) [O2(Yellow); H2(Magenta)],Stack consumption (lpm) [Air(Yellow); Fuel(Magenta)],Stack Efficiency (%)
  Current Measurement1 : spsCurrentMeasurementLib/Current Measurement  PhasorSimulation=off  OutputType=Complex  PSBequivalent=0
  Flow rate selector : Subsystem
  Flow rate selector1 : Subsystem
  Flow rate selector2 : Subsystem
  Fuel Cell Stack1 : spsFuelCellStackLib/Fuel Cell Stack  PresetModel=PEMFC - 6 kW - 45 Vdc  FcType=Proton Exchange Membrane (PEM)  Detailed=Detailed  Eoc=[65,63]  NomVI=[133.3,45]  EndVI=[225,37]  Nc=65  n=55  TOp=65  AirFr=300  SuppPress=[1.5,1]  Comp=[99.95,21,1]  SignX=off  SignY=off  FlowRateH2=on  FlowRateAir=off  SystemTemp=off  SystemPH2=off  SystemPAir=off  FCDyn=off  FC_tau=0  Peak_O2=80  V_Under=10
      settings: LibrarySourceBlock=electricdrivelib/Extra Sources/Fuel Cell Stack
  Fuel Cell Stack2 : spsFuelCellStackLib/Fuel Cell Stack  PresetModel=PEMFC - 6 kW - 45 Vdc  FcType=Proton Exchange Membrane (PEM)  Detailed=Detailed  Eoc=[65,63]  NomVI=[133.3,45]  EndVI=[225,37]  Nc=65  n=55  TOp=65  AirFr=300  SuppPress=[1.5,1]  Comp=[99.95,21,1]  SignX=off  SignY=off  FlowRateH2=on  FlowRateAir=off  SystemTemp=off  SystemPH2=off  SystemPAir=off  FCDyn=off  FC_tau=0  Peak_O2=80  V_Under=10
      settings: LibrarySourceBlock=electricdrivelib/Extra Sources/Fuel Cell Stack
  Fuel Cell Stack3 : spsFuelCellStackLib/Fuel Cell Stack  PresetModel=PEMFC - 6 kW - 45 Vdc  FcType=Proton Exchange Membrane (PEM)  Detailed=Detailed  Eoc=[65,63]  NomVI=[133.3,45]  EndVI=[225,37]  Nc=65  n=55  TOp=65  AirFr=300  SuppPress=[1.5,1]  Comp=[99.95,21,1]  SignX=off  SignY=off  FlowRateH2=on  FlowRateAir=off  SystemTemp=off  SystemPH2=off  SystemPAir=off  FCDyn=off  FC_tau=0  Peak_O2=80  V_Under=10
      settings: LibrarySourceBlock=electricdrivelib/Extra Sources/Fuel Cell Stack
  MATLAB Function : MATLAB Function  TreatAsAtomicUnit=on
  MATLAB Function1 : MATLAB Function  TreatAsAtomicUnit=on
  MATLAB Function2 : MATLAB Function  TreatAsAtomicUnit=on
  More Info : Subsystem
      settings: OpenFcn=showdemo(bdroot(gcb))
      mask Display: disp('?')
  Mux : Mux  Inputs=3
  Mux1 : Mux  Inputs=3
  Mux2 : Mux  Inputs=3
  Ramp1 : simulink/Sources/Ramp  slope=100  start=0.1  InitialOutput=0
  Ramp2 : simulink/Sources/Ramp  slope=100  start=0.1  InitialOutput=0
  Ramp3 : simulink/Sources/Ramp  slope=100  start=0.1  InitialOutput=0
  Saturation1 : Saturate  UpperLimit=48.9  LowerLimit=35  RndMeth=Nearest
  Saturation2 : Saturate  UpperLimit=48.9  LowerLimit=35  RndMeth=Nearest
  Saturation3 : Saturate  UpperLimit=48.9  LowerLimit=35  RndMeth=Nearest
  Scope{,1,3..9,11..17,19..24} (22 alike) : Scope
  Scope10 : Scope  NumInputPorts=2
  Scope18 : Scope  NumInputPorts=2
  Scope2 : Scope  NumInputPorts=4
  Series RLC Branch : spsSeriesRLCBranchLib/Series RLC Branch  LConnTagsString=__new0  RConnTagsString=__new0  BranchType=R  Resistance=100*100/6000  Inductance=100*100/6000  SetiL0=off  InitialCurrent=0  Capacitance=1e-6  Setx0=off  InitialVoltage=0  Measurements=None
  Series RLC Branch1 : spsSeriesRLCBranchLib/Series RLC Branch  LConnTagsString=__new0  RConnTagsString=__new0  BranchType=R  Resistance=100*100/6000  Inductance=100*100/6000  SetiL0=off  InitialCurrent=0  Capacitance=1e-6  Setx0=off  InitialVoltage=0  Measurements=None
  Series RLC Branch2 : spsSeriesRLCBranchLib/Series RLC Branch  LConnTagsString=__new0  RConnTagsString=__new0  BranchType=R  Resistance=100*100/6000  Inductance=100*100/6000  SetiL0=off  InitialCurrent=0  Capacitance=1e-6  Setx0=off  InitialVoltage=0  Measurements=None
  Switch : Switch  Criteria=u2 > Threshold  SaturateOnIntegerOverflow=off  InputSameDT=off
  Switch1 : Switch  Criteria=u2 > Threshold  SaturateOnIntegerOverflow=off  InputSameDT=off
  Switch2 : Switch  Criteria=u2 > Threshold  SaturateOnIntegerOverflow=off  InputSameDT=off
  Voltage Measurement1 : spsVoltageMeasurementLib/Voltage Measurement  PhasorSimulation=off  OutputType=Complex  PSBequivalent=0
  fuel cell power : Product  RndMeth=Zero
  fuel cell power1 : Product  RndMeth=Zero
  fuel cell power2 : Product  RndMeth=Zero
  powergui : spspowerguiLib/powergui  SimulationMode=Continuous  SampleTime=1e-6  frequency=60  Iterations=50  frequencyindice=0  Pbase=100e6  ErrMax=1e-4  UnitsV=kV  UnitsW=MW  buscounter=0  FunctionMessages=off  echomessages=off  EnableUseOfTLC=off  CurrentSourceSwitches=off  DisableSnubberDevices=off  DisableRonSwitches=off  DisableVfSwitches=off  DisplayEquations=off  AutomaticDiscreteSolvers=off  SolverType=Tustin  Interpol=off  ExternalGateDelay=off  methode=off  Ts=0  x0status=blocks  SPID=off  SwTol=0  HookPort=off  NonlinearTolerance=1e-4  nMaxIteration=100  ContinueOnMaxIteration=off  RestoreLinks=warning  ResistiveCurrentMeasurement=off  Frange=[0:2:500]  Ylog=off  Xlog=on  ShowGrid=off  save=off  variable=ZData  structure=0  ZoomFFT=on  StartTime=0.0  cycles=1  DisplayStyle=1  fundamental=60  FreqAxis=off  MaxFrequency=1000  frequencyindicesteady=1  RmsSteady=1  display=off
  +ve : PMIOPort  Side=Right
  " - ve" : PMIOPort  Port=2  Side=Right
  power : Outport
  wires:
  Mux/1 -> Scope6/1
  Voltage Measurement1/1 -> Scope2/3  "DC bus voltage"
  Bus Selector1/3 -> Scope4/1  "<Stack Efficiency (%)>"
  Flow rate selector/1(Ramp_Fr) -> Switch/1
  Flow rate selector/2(Sw) -> Switch/2
  fuel cell power/1 -> Add/1, Mux/1, Scope/1
  Flow rate selector/3(Fr_reg_out) -> Switch/3
  Fuel Cell Stack3/1 -> Bus Selector/1, Bus Selector1/1
  Saturation2/1 -> Fuel Cell Stack3/1, Scope1/1  "Fuel flow rate (lpm)"
  Switch/1 -> Scope7/1, Saturation2/1
  Ramp1/1 -> Flow rate selector/1(ramp)  "Fuel flow rate (lpm)"
  Current Measurement1/1 -> Scope2/4  "DC bus current"
  MATLAB Function/1(output) -> Flow rate selector/2(Fr_reg_in)
  Bus Selector1/2 -> Scope5/1  "<Stack consumption (lpm) [Air(Yellow); Fuel(Magenta)]>"
  Bus Selector/1 -> fuel cell power/1, Mux/2, Scope2/1  "<Voltage>"
  Bus Selector/2 -> MATLAB Function/1(fuelcell_current), fuel cell power/2, Mux/3, Scope2/2  "<Current>"
  Bus Selector1/1 -> Scope3/1  "<Utilization (%) [O2(Yellow); H2(Magenta)]>"
  Ramp2/1 -> Flow rate selector1/1(ramp)  "Fuel flow rate (lpm)"
  Bus Selector2/2 -> MATLAB Function1/1(fuelcell_current), fuel cell power1/2, Mux1/3, Scope10/2  "<Current>"
  Fuel Cell Stack1/1 -> Bus Selector2/1, Bus Selector3/1
  fuel cell power1/1 -> Mux1/1, Add/2, Scope8/1
  Bus Selector3/3 -> Scope12/1  "<Stack Efficiency (%)>"
  Bus Selector2/1 -> fuel cell power1/1, Mux1/2, Scope10/1  "<Voltage>"
  Flow rate selector1/3(Fr_reg_out) -> Switch1/3
  Switch1/1 -> Scope15/1, Saturation1/1
  MATLAB Function1/1(output) -> Flow rate selector1/2(Fr_reg_in)
  Saturation1/1 -> Scope9/1, Fuel Cell Stack1/1  "Fuel flow rate (lpm)"
  Flow rate selector1/1(Ramp_Fr) -> Switch1/1
  Bus Selector3/2 -> Scope13/1  "<Stack consumption (lpm) [Air(Yellow); Fuel(Magenta)]>"
  Flow rate selector1/2(Sw) -> Switch1/2
  Bus Selector3/1 -> Scope11/1  "<Utilization (%) [O2(Yellow); H2(Magenta)]>"
  Mux1/1 -> Scope14/1
  Ramp3/1 -> Flow rate selector2/1(ramp)  "Fuel flow rate (lpm)"
  Bus Selector4/2 -> MATLAB Function2/1(fuelcell_current), fuel cell power2/2, Mux2/3, Scope18/2  "<Current>"
  Fuel Cell Stack2/1 -> Bus Selector4/1, Bus Selector5/1
  fuel cell power2/1 -> Mux2/1, Add/3, Scope16/1
  Bus Selector5/3 -> Scope20/1  "<Stack Efficiency (%)>"
  Bus Selector4/1 -> fuel cell power2/1, Mux2/2, Scope18/1  "<Voltage>"
  Flow rate selector2/3(Fr_reg_out) -> Switch2/3
  Switch2/1 -> Scope23/1, Saturation3/1
  MATLAB Function2/1(output) -> Flow rate selector2/2(Fr_reg_in)
  Saturation3/1 -> Scope17/1, Fuel Cell Stack2/1  "Fuel flow rate (lpm)"
  Flow rate selector2/1(Ramp_Fr) -> Switch2/1
  Bus Selector5/2 -> Scope21/1  "<Stack consumption (lpm) [Air(Yellow); Fuel(Magenta)]>"
  Flow rate selector2/2(Sw) -> Switch2/2
  Bus Selector5/1 -> Scope19/1  "<Utilization (%) [O2(Yellow); H2(Magenta)]>"
  Mux2/1 -> Scope22/1
  Add/1 -> Scope24/1, power/1
  connections:
  100Vdc Boost DC/DC Converter (average value)1/LConn2 -- Fuel Cell Stack1/RConn2
  100Vdc Boost DC/DC Converter (average value)/RConn1 -- Current Measurement1/LConn1 -- Voltage Measurement1/LConn1
  100Vdc Boost DC/DC Converter (average value)1/LConn1 -- Fuel Cell Stack1/RConn1
  Series RLC Branch2/RConn1 -- " - ve"/RConn1 -- 100Vdc Boost DC/DC Converter (average value)/RConn2 -- Voltage Measurement1/LConn2 -- Series RLC Branch/RConn1 -- 100Vdc Boost DC/DC Converter (average value)1/RConn2 -- Series RLC Branch1/RConn1 -- 100Vdc Boost DC/DC Converter (average value)2/RConn2
  Fuel Cell Stack3/RConn2 -- 100Vdc Boost DC/DC Converter (average value)/LConn2
  Fuel Cell Stack3/RConn1 -- 100Vdc Boost DC/DC Converter (average value)/LConn1
  Series RLC Branch/LConn1 -- Current Measurement1/RConn1 -- 100Vdc Boost DC/DC Converter (average value)2/RConn1 -- Series RLC Branch2/LConn1 -- 100Vdc Boost DC/DC Converter (average value)1/RConn1 -- Series RLC Branch1/LConn1 -- +ve/RConn1
  100Vdc Boost DC/DC Converter (average value)2/LConn1 -- Fuel Cell Stack2/RConn1
  100Vdc Boost DC/DC Converter (average value)2/LConn2 -- Fuel Cell Stack2/RConn2

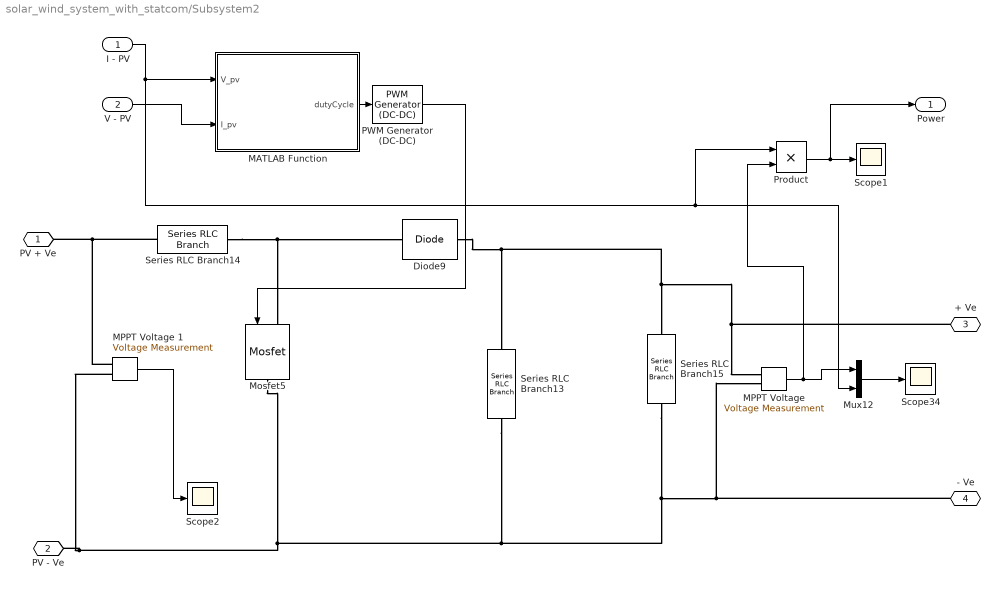
== system solar_wind_system_with_statcom/Subsystem2 ==
  I - PV : Inport
  V - PV : Inport  Port=2
  Diode9 : spsDiodeLib/Diode  Ron=0.001  Lon=0  Vf=0.8  IC=0  UseSnubber=off  Rs=500  Cs=250e-9  Measurements=off
  MATLAB Function : MATLAB Function  TreatAsAtomicUnit=on
  "MPPT Voltage " : spsVoltageMeasurementLib/Voltage Measurement  PhasorSimulation=off  OutputType=Complex  PSBequivalent=0
  MPPT Voltage 1 : spsVoltageMeasurementLib/Voltage Measurement  PhasorSimulation=off  OutputType=Complex  PSBequivalent=0
  Mosfet5 : spsMosfetLib/Mosfet  Ron=0.1  Lon=0  Rd=0.01  Vfd=0  IC=0  Rs=1e5  Cs=inf  Measurements=off
  Mux12 : Mux  Inputs=2
  PWM Generator (DC-DC) : spsPWMGeneratorDCDCLib/PWM Generator (DC-DC)  Fsw=5000  Ts=0
  Product : Product
  Scope1 : Scope
  Scope2 : Scope
  Scope34 : Scope
  Series RLC Branch13 : spsSeriesRLCBranchLib/Series RLC Branch  LConnTagsString=__new0  RConnTagsString=__new0  BranchType=C  Resistance=1  Inductance=1e-3  SetiL0=off  InitialCurrent=0  Capacitance=550e-6  Setx0=off  InitialVoltage=0  Measurements=None
  Series RLC Branch14 : spsSeriesRLCBranchLib/Series RLC Branch  LConnTagsString=__new0  RConnTagsString=__new0  BranchType=L  Resistance=1  Inductance=0.05e-2  SetiL0=off  InitialCurrent=0  Capacitance=1e-6  Setx0=off  InitialVoltage=0  Measurements=None
  Series RLC Branch15 : spsSeriesRLCBranchLib/Series RLC Branch  LConnTagsString=__new0  RConnTagsString=__new0  BranchType=R  Resistance=20  Inductance=1e-3  SetiL0=off  InitialCurrent=0  Capacitance=1e-6  Setx0=off  InitialVoltage=0  Measurements=None
  PV + Ve : PMIOPort  Side=Left
  PV - Ve : PMIOPort  Port=2  Side=Left
  + Ve : PMIOPort  Port=3  Side=Right
  - Ve : PMIOPort  Port=4  Side=Right
  Power : Outport
  wires:
  MPPT Voltage 1/1 -> Scope2/1
  Mux12/1 -> Scope34/1
  "MPPT Voltage "/1 -> Product/2, Mux12/1
  I - PV/1 -> MATLAB Function/1(V_pv), Product/1, Mux12/2
  PWM Generator (DC-DC)/1 -> Mosfet5/1
  V - PV/1 -> MATLAB Function/2(I_pv)
  Product/1 -> Power/1, Scope1/1
  MATLAB Function/1(dutyCycle) -> PWM Generator (DC-DC)/1
  connections:
  MPPT Voltage 1/LConn1 -- Series RLC Branch14/LConn1 -- PV + Ve/RConn1
  MPPT Voltage 1/LConn2 -- PV - Ve/RConn1 -- Series RLC Branch13/RConn1 -- - Ve/RConn1 -- "MPPT Voltage "/LConn2 -- Series RLC Branch15/RConn1 -- Mosfet5/RConn1
  + Ve/RConn1 -- Series RLC Branch13/LConn1 -- Diode9/RConn1 -- Series RLC Branch15/LConn1 -- "MPPT Voltage "/LConn1
  Series RLC Branch14/RConn1 -- Diode9/LConn1 -- Mosfet5/LConn1

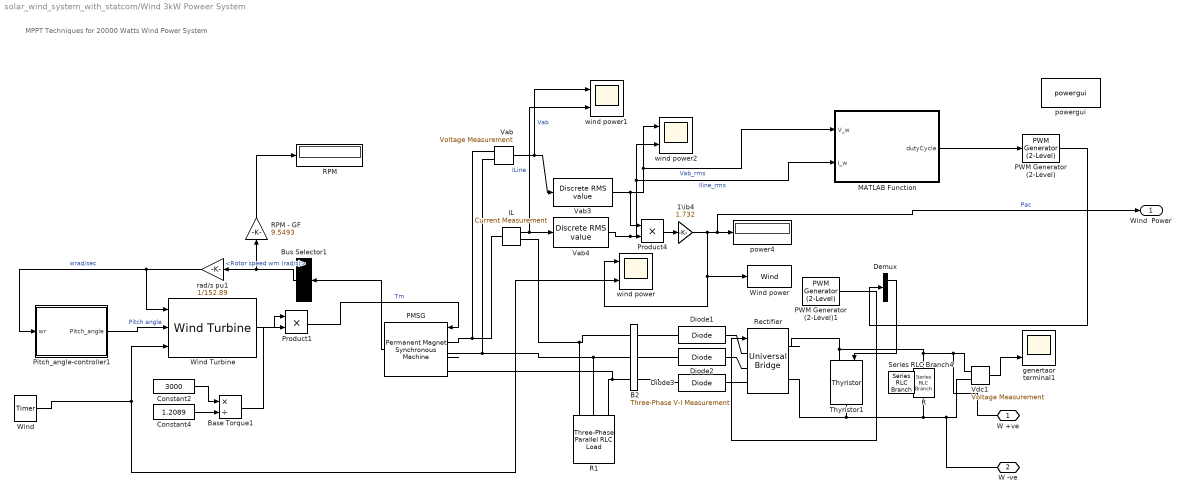
== system solar_wind_system_with_statcom/Wind 3kW Poweer System ==
  note: MPPT Techniques for 20000 Watts Wind Power System
  1\ib4 : Gain  Gain=1.732  SaturateOnIntegerOverflow=on  OutDataTypeStr=Inherit: Same as input  ParamDataTypeStr=Inherit: Same as input
  "B2 " : spsThreePhaseVIMeasurementLib/Three-Phase V-I Measurement  VoltageMeasurement=no  SetLabelV=on  LabelV=Vabc_B2  Vpu=off  VpuLL=off  CurrentMeasurement=no  SetLabelI=on  LabelI=Iabc_B2  Ipu=off  Pbase=100e6  Vbase=500e3  OutputType=Magnitude  PhasorSimulation=off  PSBequivalent=0
  Base Torque1 : Product  Inputs=*/  RndMeth=Zero
  Bus Selector1 : BusSelector  OutputSignals=Rotor speed wm (rad/s)
  Constant2 : Constant  Value=3000
  Constant4 : Constant  Value=1.2089
  Demux : Demux  Outputs=2
  Diode1 : spsDiodeLib/Diode  Ron=0.001  Lon=0  Vf=0.8  IC=0  UseSnubber=off  Rs=500  Cs=250e-9  Measurements=off
  Diode2 : spsDiodeLib/Diode  Ron=0.001  Lon=0  Vf=0.8  IC=0  UseSnubber=off  Rs=500  Cs=250e-9  Measurements=off
  Diode3 : spsDiodeLib/Diode  Ron=0.001  Lon=0  Vf=0.8  IC=0  UseSnubber=off  Rs=500  Cs=250e-9  Measurements=off
  IL : spsCurrentMeasurementLib/Current Measurement  PhasorSimulation=off  OutputType=Complex  PSBequivalent=0
  MATLAB Function : MATLAB Function  TreatAsAtomicUnit=on
  PMSG : spsPermanentMagnetSynchronousMachineLib/Permanent Magnet Synchronous Machine  NbPhases=3  FluxDistribution=Sinusoidal  RotorType=Round  MechanicalLoad=Torque Tm  PresetModel=No  ShowDetailedParameters=on  MeasurementBus=off  Resistance=0.0918  Inductance=8.5e-3  dqInductances=[0.0082 0.0082]  La=0.000975  MachineConstant=Flux linkage established by magnets (V.s)  Flux=0.1688  VoltageCst=122.4677  TorqueCst=1.0128  Flat=120  Mechanical=[0.003945 0.0004924 4 0]  PolePairs=4  InitialConditions=[0,0, 0,0]  InitialConditions5ph=[0 0 0 0 0 0]  RefAngle=90 degrees behind phase A axis (modified Park)  IterativeDiscreteModel=Trapezoidal non iterative  TsBlock=-1  TsPowergui=0
  PWM Generator (2-Level) : spsPWMGenerator2LevelLib/PWM Generator (2-Level)  ModulatorType=Single-phase half-bridge (2 pulses)  ModulatorMode=Unsynchronized  Fc=3000  Pc=90  nF=27  MinMax="[ -1  1 ]"  SamplingTechnique=Natural  ModulatingSignals=off  m=0.8  Freq=60  Phase=0  Ts=0  ShowCarrierOutport=off
  PWM Generator (2-Level)1 : spsPWMGenerator2LevelLib/PWM Generator (2-Level)  ModulatorType=Three-phase bridge (6 pulses)  ModulatorMode=Unsynchronized  Fc=27*60  Pc=90  nF=27  MinMax="[ -1  1 ]"  SamplingTechnique=Natural  ModulatingSignals=on  m=0.7  Freq=50  Phase=0  Ts=0  ShowCarrierOutport=off
  Pitch_angle-controller1 : Subsystem
  Product1 : Product  RndMeth=Zero
  Product4 : Product  RndMeth=Zero
  R : spsSeriesRLCBranchLib/Series RLC Branch  LConnTagsString=__new0  RConnTagsString=__new0  BranchType=R  Resistance=20  Inductance=1e-3  SetiL0=off  InitialCurrent=0  Capacitance=1e-6  Setx0=off  InitialVoltage=0  Measurements=None
  "R1 " : spsThreePhaseParallelRLCLoadLib/Three-Phase Parallel RLC Load  LConnTagsString=A|B|C  Configuration=Y (grounded)  NominalVoltage=220  Vabc=[1e3 1e3 1e3]  Vabcp=[1e3 1e3 1e3]  NominalFrequency=50  UnbalancedPower=off  ActivePower=24000  InductivePower=0  CapacitivePower=0  Pabc=[9e3 9e3 9e3]  QLabc=[100 90 110]  QCabc=[100 90 110]  Pabcp=[10e3 9e3 11e3]  QLabcp=[100 90 110]  QCabcp=[100 90 110]  Measurements=None  LoadType=constant Z
  "RPM " : Display
  RPM - GF : Gain  Gain=9.5493  SaturateOnIntegerOverflow=on  OutDataTypeStr=Inherit: Same as input  ParamDataTypeStr=Inherit: Same as input
  Rectifier : spsUniversalBridgeLib/Universal Bridge  Arms=3  SnubberResistance=100  SnubberCapacitance=0.1e-6  Device=IGBT / Diodes  Ron=1e-3  Lon=0  ForwardVoltages="[  100  100  ]"  ForwardVoltage=.8  GTOparameters=[ 10e-6 , 20e-6 ]  IGBTparameters=[ 1e-6 , 2e-6 ]  Measurements=Device currents  Measurements_2=None  converterType=Rectifier
      settings: AttributesFormatString=\n
  Series RLC Branch4 : spsSeriesRLCBranchLib/Series RLC Branch  LConnTagsString=__new0  RConnTagsString=__new0  BranchType=C  Resistance=R  Inductance=1e-3  SetiL0=off  InitialCurrent=0  Capacitance=470e-5  Setx0=off  InitialVoltage=0  Measurements=Branch voltage and current
  Thyristor1 : spsThyristorLib/Thyristor  Ron=0.001  Lon=0  Vf=220  IC=0  Rs=500  Cs=250e-9  Measurements=off
  Vab : spsVoltageMeasurementLib/Voltage Measurement  PhasorSimulation=off  OutputType=Complex  PSBequivalent=0
  Vab3 : powerlib_extras/Discrete Measurements/Discrete  RMS value  Freq=50  Mag_Init=0  Ts=20e-6
  Vab4 : powerlib_extras/Discrete Measurements/Discrete  RMS value  Freq=50  Mag_Init=0  Ts=20e-6
  Vdc1 : spsVoltageMeasurementLib/Voltage Measurement  Tag=PoWeRsYsTeMmEaSuReMeNt  PhasorSimulation=off  OutputType=Magnitude  PSBequivalent=0
  "Wind " : powerlib_extras/Control  Blocks/Timer  t=[0 0.05 0.1 0.15 0.2 ]  e=[5 7 11 12 12]
  Wind Turbine : spsWindTurbineLib/Wind Turbine  Pnom=20000  Pelec_base=20000/0.9  wind_base=12  P_wind_base=0.73  speed_nom=1.2  pitch_angle=0  c1_c6="[0.51763          116          0.4            5           21     0.006795]"  cp_nom=0.48  lambda_nom=8.1
  Wind power : ToWorkspace  VariableName=Wind  SaveFormat=Timeseries  SampleTime=-1
  genertaor terminal1 : Scope  NumInputPorts=2
  power4 : Display
      settings: SampleTime=1e-3
  powergui : spspowerguiLib/powergui  Priority=1  SimulationMode=Continuous  SampleTime=50e-6  frequency=60  Iterations=50  frequencyindice=0  Pbase=100e6  ErrMax=1e-4  UnitsV=kV  UnitsW=MW  buscounter=0  FunctionMessages=off  echomessages=off  EnableUseOfTLC=off  CurrentSourceSwitches=off  DisableSnubberDevices=off  DisableRonSwitches=off  DisableVfSwitches=off  DisplayEquations=off  AutomaticDiscreteSolvers=off  SolverType=Tustin/Backward Euler (TBE)  Interpol=off  ExternalGateDelay=off  methode=off  Ts=100  x0status=blocks  SPID=on  SwTol=0  HookPort=off  NonlinearTolerance=1e-4  nMaxIteration=100  ContinueOnMaxIteration=off  RestoreLinks=warning  ResistiveCurrentMeasurement=off  Frange=[0:2:500]  Ylog=off  Xlog=on  ShowGrid=off  save=off  variable=ZData  structure=0  ZoomFFT=off  StartTime=0.0  cycles=1  DisplayStyle=1  fundamental=60  FreqAxis=off  MaxFrequency=1000  frequencyindicesteady=1  RmsSteady=1  display=off
  rad/s pu1 : Gain  Gain=1/152.89  SaturateOnIntegerOverflow=on  OutDataTypeStr=Inherit: Same as input  ParamDataTypeStr=Inherit: Same as input
  wind power : Scope  NumInputPorts=2
  wind power1 : Scope  NumInputPorts=2
  wind power2 : Scope  NumInputPorts=2
  W +ve : PMIOPort  Side=Right
  W -ve : PMIOPort  Port=2  Side=Right
  Wind  Power : Outport
  wires:
  PMSG/1 -> Bus Selector1/1
  rad/s pu1/1 -> Wind Turbine/1, Pitch_angle-controller1/1(wr)  "wrad/sec"
  Product1/1 -> PMSG/1  "Tm"
  Vab3/1 -> Product4/1, MATLAB Function/1(V_w), wind power2/1  "Vab_rms"
  Product4/1 -> 1\ib4/1
  Bus Selector1/1 -> RPM - GF/1, rad/s pu1/1  "<Rotor speed wm (rad/s)>"
  1\ib4/1 -> Wind  Power/1, power4/1, Wind power/1, wind power/1  "Pac"
  Vab/1 -> wind power1/1, Vab3/1  "Vab"
  Vdc1/1 -> genertaor terminal1/2
  "Wind "/1 -> Wind Turbine/3, wind power/2
  Vab4/1 -> MATLAB Function/2(I_w), wind power2/2, Product4/2  "Iline_rms"
  Pitch_angle-controller1/1(Pitch_angle) -> Wind Turbine/2  "Pitch angle"
  Constant2/1 -> Base Torque1/1
  Base Torque1/1 -> Product1/2
  IL/1 -> wind power1/2, Vab4/1  "ILine"
  Wind Turbine/1 -> Product1/1
  RPM - GF/1 -> "RPM "/1
  Constant4/1 -> Base Torque1/2
  PWM Generator (2-Level)/1 -> Demux/1
  Demux/1 -> Thyristor1/1
  PWM Generator (2-Level)1/1 -> Rectifier/1
  MATLAB Function/1(dutyCycle) -> PWM Generator (2-Level)/1
  connections:
  W +ve/RConn1 -- Vdc1/LConn1 -- R/LConn1 -- Rectifier/RConn1 -- Thyristor1/LConn1
  Rectifier/RConn2 -- Vdc1/LConn2 -- W -ve/RConn1 -- R/RConn1 -- Thyristor1/RConn1
  Diode2/RConn1 -- Rectifier/LConn2
  IL/RConn1 -- "B2 "/LConn1 -- "R1 "/LConn1
  PMSG/LConn2 -- Vab/LConn2 -- "B2 "/LConn2 -- "R1 "/LConn2
  "B2 "/RConn3 -- Diode3/LConn1
  PMSG/LConn1 -- Vab/LConn1 -- IL/LConn1
  "B2 "/LConn3 -- PMSG/LConn3 -- "R1 "/LConn3
  Diode1/RConn1 -- Rectifier/LConn1
  Diode1/LConn1 -- "B2 "/RConn1
  Diode3/RConn1 -- Rectifier/LConn3
  Diode2/LConn1 -- "B2 "/RConn2
